simulink model "exp2"  (R2020b)
settings: Solver=VariableStepAuto  StartTime=0.0  StopTime=150  RelTol=1e-3
libraries: simulink x2
settings Model: Creator=suryanshshukla  LastModifiedBy=suryanshshukla

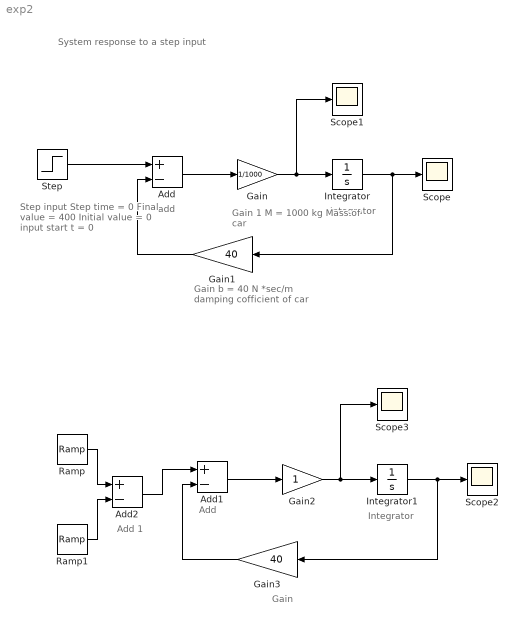
== system exp2 ==
  note: Integrator
  note: add
  note: Gain
      | b = 40 N *sec/m
      | damping cofficient of car
  note: Gain 1
      | M = 1000 kg
      | Mass of car
  note: Step input
      | Step time = 0
      | Final value = 400
      | Initial value = 0
      | input start t = 0
  note: Integrator
  note: Gain
  note: Add
  note: Add 1
  note: System response to a step input
  Add : Sum  Inputs=+-
  Add1 : Sum  Inputs=+-
  Add2 : Sum  Inputs=+-
  Gain : Gain  Gain=1/1000
  Gain1 : Gain  Gain=40
  Gain2 : Gain
  Gain3 : Gain  Gain=40
  Integrator : Integrator
  Integrator1 : Integrator
  Ramp : simulink/Sources/Ramp  slope=1  start=0  InitialOutput=0
  Ramp1 : simulink/Sources/Ramp  slope=1  start=0  InitialOutput=0
  Scope{,1..3} (4 alike) : Scope
  Step : Step  Time=0  After=400  SampleTime=0
  wires:
  Step/1 -> Add/1
  Add/1 -> Gain/1
  Gain1/1 -> Add/2
  Integrator/1 -> Gain1/1, Scope/1
  Gain/1 -> Scope1/1, Integrator/1
  Integrator1/1 -> Gain3/1, Scope2/1
  Gain3/1 -> Add1/2
  Gain2/1 -> Scope3/1, Integrator1/1
  Add1/1 -> Gain2/1
  Add2/1 -> Add1/1
  Ramp/1 -> Add2/1
  Ramp1/1 -> Add2/2
